simulink model "PVHome"  (R2022b)
settings: Solver=FixedStepDiscrete  StartTime=0.0  StopTime=2  FixedStep=5e-6  RelTol=1e-3
undefined symbols (not defined in the file): Ion, Lithium
libraries: spsSeriesRLCBranchLib x175, spsBreakerLib x103, spsPWMGeneratorDCDCLib x94, spsThyristorLib x78, slpidlib x72, spsIGBTDiodeLib x62, spsThreePhaseVIMeasurementLib x59, spsThreePhaseBreakerLib x45, spsVoltageMeasurementLib x45, spsDiodeLib x39, spsThreePhaseParallelRLCBranchLib x38, spsMosfetLib x32
(part 13 of 16)

== system PVHome/Subsystem6/Subsystem ==
  note: this must activate when no power is available in the pv or no sufficient power available in PV
  note: Buck conv
  note: REAL GRID
  note: House Load DC to AC conversion
  note: Buck conv
  note: Buck conv
  Add{1..4} (4 alike) : Sum  Inputs=+-
  Battery1 : spsBatteryLib/Battery  BatType=Lithium-Ion  ShowTempParam=off  ThermalPreset=no  ShowAgeParam=off  NomV=60  NomQ=50  SOC=50  Batt_Tr=1  PresetModel=off  MaxQ=50  MinV=45  FullV=69.8392  Dis_rate=21.7391  R=0.012  Normal_OP=45.2174  expZone="[64.8232      2.45652]"  current=[6.5 13 32.5]  Units=Time  Tci=20  NomT=20  T2=-30  MaxQ2=4.8  FullV2=7.1  Normal_OP2=5.655  expZone2="[6.58           1]"  Rca=0.6  ti=2000  Dp=0  Neq0=0  Tsim=1e6  Ta1=25  Qeol=5.4*0.9  Reol=0.013333*1.2  Char_age=[2.3478, 3]  Dis_age=[2.3478, 10]  N1=1500  N2=10500  N3=1000  N4=1400  Ta2=45  N5=950
  Breaker{11..13,17..18,20} (6 alike) : spsBreakerLib/Breaker  InitialState=0  SwitchingTimes="[1/60  5/60]"  External=on  BreakerResistance=0.01  SnubberResistance=1e6  SnubberCapacitance=inf  Measurements=None  MoreParameters=on  NoBreakLoop=off
  Bus Creator1 : BusCreator  Inputs=3
  Bus Selector2 : BusSelector  OutputSignals=SOC (%),Current (A),Voltage (V)
  CAPACITOR 15 : spsSeriesRLCBranchLib/Series RLC Branch  LConnTagsString=__new0  RConnTagsString=__new0  BranchType=RL  Resistance=1e-4  Inductance=1e-3  SetiL0=off  InitialCurrent=0  Capacitance=100e-6  Setx0=off  InitialVoltage=0  Measurements=None
  CAPACITOR 20 : spsSeriesRLCBranchLib/Series RLC Branch  LConnTagsString=__new0  RConnTagsString=__new0  BranchType=RC  Resistance=1e-4  Inductance=5e-3  SetiL0=off  InitialCurrent=0  Capacitance=100e-6  Setx0=off  InitialVoltage=0  Measurements=None
  CAPACITOR 21 : spsSeriesRLCBranchLib/Series RLC Branch  LConnTagsString=__new0  RConnTagsString=__new0  BranchType=RC  Resistance=1e-4  Inductance=5e-3  SetiL0=off  InitialCurrent=0  Capacitance=100e-6  Setx0=off  InitialVoltage=0  Measurements=None
  CAPACITOR 22 : spsSeriesRLCBranchLib/Series RLC Branch  LConnTagsString=__new0  RConnTagsString=__new0  BranchType=RL  Resistance=1e-4  Inductance=13e-3  SetiL0=off  InitialCurrent=0  Capacitance=100e-6  Setx0=off  InitialVoltage=0  Measurements=None
  CAPACITOR 27 : spsSeriesRLCBranchLib/Series RLC Branch  LConnTagsString=__new0  RConnTagsString=__new0  BranchType=RL  Resistance=1e-4  Inductance=1e-3  SetiL0=off  InitialCurrent=0  Capacitance=100e-6  Setx0=off  InitialVoltage=0  Measurements=None
  CAPACITOR 28 : spsSeriesRLCBranchLib/Series RLC Branch  LConnTagsString=__new0  RConnTagsString=__new0  BranchType=RC  Resistance=1e-4  Inductance=5e-3  SetiL0=off  InitialCurrent=0  Capacitance=2000e-3  Setx0=off  InitialVoltage=0  Measurements=None
  CAPACITOR 29 : spsSeriesRLCBranchLib/Series RLC Branch  LConnTagsString=__new0  RConnTagsString=__new0  BranchType=RC  Resistance=1e-4  Inductance=5e-3  SetiL0=off  InitialCurrent=0  Capacitance=2000e-3  Setx0=off  InitialVoltage=0  Measurements=None
  CAPACITOR 30 : spsSeriesRLCBranchLib/Series RLC Branch  LConnTagsString=__new0  RConnTagsString=__new0  BranchType=RL  Resistance=1e-4  Inductance=1e-3  SetiL0=off  InitialCurrent=0  Capacitance=100e-6  Setx0=off  InitialVoltage=0  Measurements=None
  CAPACITOR 31 : spsSeriesRLCBranchLib/Series RLC Branch  LConnTagsString=__new0  RConnTagsString=__new0  BranchType=RC  Resistance=1e-4  Inductance=5e-3  SetiL0=off  InitialCurrent=0  Capacitance=2000e-3  Setx0=off  InitialVoltage=0  Measurements=None
  Constant7 : Constant  Value=60
  Constant9 : Constant  Value=2300
  Current Measurement4 : spsCurrentMeasurementLib/Current Measurement  PhasorSimulation=off  OutputType=Complex  PSBequivalent=0
  Data Type Conversion3 : DataTypeConversion  OutDataTypeStr=boolean  SaturateOnIntegerOverflow=off  RndMeth=Floor
  Demux1 : Demux  Outputs=2
  Diode5 : spsDiodeLib/Diode  Ron=0.001  Lon=0  Vf=0.8  IC=0  UseSnubber=0  Rs=500  Cs=250e-9  Measurements=off
  Diode7 : spsDiodeLib/Diode  Ron=0.001  Lon=0  Vf=0.8  IC=0  UseSnubber=0  Rs=500  Cs=250e-9  Measurements=off
  Discrete PID Controller1 : slpidlib/PID Controller  Controller=PI  Form=Parallel  TimeDomain=Discrete-time  UseExternalTs=off  SampleTime=1e-5  IntegratorMethod=Forward Euler  FilterMethod=Forward Euler  ControllerParametersSource=internal  P=0  I=0.01  UseKiTs=off  D=0  N=100  UseFilter=on  TunerSelectOption=Transfer Function Based (PID Tuner App)  InitialConditionSource=internal  InitialConditionForIntegrator=0  InitialConditionForFilter=0  DifferentiatorICPrevScaledInput=0  ExternalReset=none  TrackingMode=off  Kt=1  LimitOutput=on  SatLimitsSource=internal  UpperSaturationLimit=1.1  LowerSaturationLimit=-1.1  LinearizeAsGain=off  AntiWindupMode=none  Kb=1  LimitIntegrator=off  UpperIntegratorSaturationLimit=inf  LowerIntegratorSaturationLimit=-inf  POutMin=[]  POutMax=[]  IOutMin=[]  IOutMax=[]  DOutMin=[]  DOutMax=[]  NOutMin=[]  NOutMax=[]  SumOutMin=[]  SumOutMax=[]  SaturationOutMin=[]  SaturationOutMax=[]  PParamMin=[]  PParamMax=[]  IParamMin=[]  IParamMax=[]  DParamMin=[]  DParamMax=[]  NParamMin=[]  NParamMax=[]  KbParamMin=[]  KbParamMax=[]  KtParamMin=[]  KtParamMax=[]  KbOutMin=[]  KbOutMax=[]  KtOutMin=[]  KtOutMax=[]  IntegratorOutMin=[]  IntegratorOutMax=[]  FilterOutMin=[]  FilterOutMax=[]  SumI1OutMin=[]  SumI1OutMax=[]  SumI2OutMin=[]  SumI2OutMax=[]  SumI3OutMin=[]  SumI3OutMax=[]  SumI4OutMin=[]  SumI4OutMax=[]  SumDOutMin=[]  SumDOutMax=[]  DifferentiatorOutMin=[]  DifferentiatorOutMax=[]  FilterDiffOutCoefMin=[]  FilterDiffOutCoefMax=[]  ReciprocalOutMin=[]  ReciprocalOutMax=[]  SumDenOutMin=[]  SumDenOutMax=[]  SumNumOutMin=[]  SumNumOutMax=[]  DivideOutMin=[]  DivideOutMax=[]  UdiffTsProdOutMin=[]  UdiffTsProdOutMax=[]  NTsProdOutMin=[]  NTsProdOutMax=[]  UintegralTsProdOutMin=[]  UintegralTsProdOutMax=[]  UngainTsProdOutMin=[]  UngainTsProdOutMax=[]  ClampingZeroOutDataTypeStr=Inherit: Inherit via back propagation  ClampingZeroOutMin=[]  ClampingZeroOutMax=[]  FilterDenConstantOutDataTypeStr=Inherit: Inherit via back propagation  FilterDenConstantOutMin=[]  FilterDenConstantOutMax=[]  PCopyOutDataTypeStr=Inherit: Inherit via back propagation  PCopyOutMin=[]  PCopyOutMax=[]  NCopyOutDataTypeStr=Inherit: Inherit via back propagation  NCopyOutMin=[]  NCopyOutMax=[]  IntegratorContinuousStateAttributes=''  IntegratorStateMustResolveToSignalObject=off  IntegratorRTWStateStorageClass=Auto  FilterContinuousStateAttributes=''  FilterStateMustResolveToSignalObject=off  FilterRTWStateStorageClass=Auto  ParallelPVariant=InternalParameters  IdealPVariant=Disabled  IVariant=InternalParameters  DVariant=Disabled  IntegratorVariant=Discrete  SatVariant=Enabled  AWVariant=Passthrough  PCopyVariant=Disabled  TRVariant=Disabled  FdbkBlocksVariant=Forward  IdealPFdbkVariant=Disabled  SatFdbkVariant=Disabled  DerivativeFilterVariant=Disabled  NVariant=Disabled  NCopyVariant=Disabled_SignalSpec  FilterICVariant=Disabled  IntegratorICVariant=InternalICs  ExternalResetVariant=Disabled  TRSumVariant=Passthrough  SumFdbkVariant=Disabled  SumVariant=Sum_PI  TsampFilterVariant=InternalTs  TsampNgainVariant=Passthrough  TsampIntegralVariant=Passthrough  ExternalSaturationOutDataTypeStr=Inherit: Same as second input
      settings: LibrarySourceBlock=simulink/Discrete/Discrete PID Controller
  Discrete PID Controller2 : slpidlib/PID Controller  Controller=PI  Form=Parallel  TimeDomain=Discrete-time  UseExternalTs=off  SampleTime=1e-5  IntegratorMethod=Forward Euler  FilterMethod=Forward Euler  ControllerParametersSource=internal  P=0.01  I=1  UseKiTs=off  D=0  N=100  UseFilter=on  TunerSelectOption=Transfer Function Based (PID Tuner App)  InitialConditionSource=internal  InitialConditionForIntegrator=0  InitialConditionForFilter=0  DifferentiatorICPrevScaledInput=0  ExternalReset=none  TrackingMode=off  Kt=1  LimitOutput=on  SatLimitsSource=internal  UpperSaturationLimit=1.1  LowerSaturationLimit=-1.1  LinearizeAsGain=off  AntiWindupMode=none  Kb=1  LimitIntegrator=off  UpperIntegratorSaturationLimit=inf  LowerIntegratorSaturationLimit=-inf  POutMin=[]  POutMax=[]  IOutMin=[]  IOutMax=[]  DOutMin=[]  DOutMax=[]  NOutMin=[]  NOutMax=[]  SumOutMin=[]  SumOutMax=[]  SaturationOutMin=[]  SaturationOutMax=[]  PParamMin=[]  PParamMax=[]  IParamMin=[]  IParamMax=[]  DParamMin=[]  DParamMax=[]  NParamMin=[]  NParamMax=[]  KbParamMin=[]  KbParamMax=[]  KtParamMin=[]  KtParamMax=[]  KbOutMin=[]  KbOutMax=[]  KtOutMin=[]  KtOutMax=[]  IntegratorOutMin=[]  IntegratorOutMax=[]  FilterOutMin=[]  FilterOutMax=[]  SumI1OutMin=[]  SumI1OutMax=[]  SumI2OutMin=[]  SumI2OutMax=[]  SumI3OutMin=[]  SumI3OutMax=[]  SumI4OutMin=[]  SumI4OutMax=[]  SumDOutMin=[]  SumDOutMax=[]  DifferentiatorOutMin=[]  DifferentiatorOutMax=[]  FilterDiffOutCoefMin=[]  FilterDiffOutCoefMax=[]  ReciprocalOutMin=[]  ReciprocalOutMax=[]  SumDenOutMin=[]  SumDenOutMax=[]  SumNumOutMin=[]  SumNumOutMax=[]  DivideOutMin=[]  DivideOutMax=[]  UdiffTsProdOutMin=[]  UdiffTsProdOutMax=[]  NTsProdOutMin=[]  NTsProdOutMax=[]  UintegralTsProdOutMin=[]  UintegralTsProdOutMax=[]  UngainTsProdOutMin=[]  UngainTsProdOutMax=[]  ClampingZeroOutDataTypeStr=Inherit: Inherit via back propagation  ClampingZeroOutMin=[]  ClampingZeroOutMax=[]  FilterDenConstantOutDataTypeStr=Inherit: Inherit via back propagation  FilterDenConstantOutMin=[]  FilterDenConstantOutMax=[]  PCopyOutDataTypeStr=Inherit: Inherit via back propagation  PCopyOutMin=[]  PCopyOutMax=[]  NCopyOutDataTypeStr=Inherit: Inherit via back propagation  NCopyOutMin=[]  NCopyOutMax=[]  IntegratorContinuousStateAttributes=''  IntegratorStateMustResolveToSignalObject=off  IntegratorRTWStateStorageClass=Auto  FilterContinuousStateAttributes=''  FilterStateMustResolveToSignalObject=off  FilterRTWStateStorageClass=Auto  ParallelPVariant=InternalParameters  IdealPVariant=Disabled  IVariant=InternalParameters  DVariant=Disabled  IntegratorVariant=Discrete  SatVariant=Enabled  AWVariant=Passthrough  PCopyVariant=Disabled  TRVariant=Disabled  FdbkBlocksVariant=Forward  IdealPFdbkVariant=Disabled  SatFdbkVariant=Disabled  DerivativeFilterVariant=Disabled  NVariant=Disabled  NCopyVariant=Disabled_SignalSpec  FilterICVariant=Disabled  IntegratorICVariant=InternalICs  ExternalResetVariant=Disabled  TRSumVariant=Passthrough  SumFdbkVariant=Disabled  SumVariant=Sum_PI  TsampFilterVariant=InternalTs  TsampNgainVariant=Passthrough  TsampIntegralVariant=Passthrough  ExternalSaturationOutDataTypeStr=Inherit: Same as second input
      settings: LibrarySourceBlock=simulink/Discrete/Discrete PID Controller
  Discrete PID Controller3 : slpidlib/PID Controller  Controller=PI  Form=Parallel  TimeDomain=Discrete-time  UseExternalTs=off  SampleTime=1e-5  IntegratorMethod=Forward Euler  FilterMethod=Forward Euler  ControllerParametersSource=internal  P=0  I=0.01  UseKiTs=off  D=0  N=100  UseFilter=on  TunerSelectOption=Transfer Function Based (PID Tuner App)  InitialConditionSource=internal  InitialConditionForIntegrator=0  InitialConditionForFilter=0  DifferentiatorICPrevScaledInput=0  ExternalReset=none  TrackingMode=off  Kt=1  LimitOutput=on  SatLimitsSource=internal  UpperSaturationLimit=1.1  LowerSaturationLimit=-1.1  LinearizeAsGain=off  AntiWindupMode=none  Kb=1  LimitIntegrator=off  UpperIntegratorSaturationLimit=inf  LowerIntegratorSaturationLimit=-inf  POutMin=[]  POutMax=[]  IOutMin=[]  IOutMax=[]  DOutMin=[]  DOutMax=[]  NOutMin=[]  NOutMax=[]  SumOutMin=[]  SumOutMax=[]  SaturationOutMin=[]  SaturationOutMax=[]  PParamMin=[]  PParamMax=[]  IParamMin=[]  IParamMax=[]  DParamMin=[]  DParamMax=[]  NParamMin=[]  NParamMax=[]  KbParamMin=[]  KbParamMax=[]  KtParamMin=[]  KtParamMax=[]  KbOutMin=[]  KbOutMax=[]  KtOutMin=[]  KtOutMax=[]  IntegratorOutMin=[]  IntegratorOutMax=[]  FilterOutMin=[]  FilterOutMax=[]  SumI1OutMin=[]  SumI1OutMax=[]  SumI2OutMin=[]  SumI2OutMax=[]  SumI3OutMin=[]  SumI3OutMax=[]  SumI4OutMin=[]  SumI4OutMax=[]  SumDOutMin=[]  SumDOutMax=[]  DifferentiatorOutMin=[]  DifferentiatorOutMax=[]  FilterDiffOutCoefMin=[]  FilterDiffOutCoefMax=[]  ReciprocalOutMin=[]  ReciprocalOutMax=[]  SumDenOutMin=[]  SumDenOutMax=[]  SumNumOutMin=[]  SumNumOutMax=[]  DivideOutMin=[]  DivideOutMax=[]  UdiffTsProdOutMin=[]  UdiffTsProdOutMax=[]  NTsProdOutMin=[]  NTsProdOutMax=[]  UintegralTsProdOutMin=[]  UintegralTsProdOutMax=[]  UngainTsProdOutMin=[]  UngainTsProdOutMax=[]  ClampingZeroOutDataTypeStr=Inherit: Inherit via back propagation  ClampingZeroOutMin=[]  ClampingZeroOutMax=[]  FilterDenConstantOutDataTypeStr=Inherit: Inherit via back propagation  FilterDenConstantOutMin=[]  FilterDenConstantOutMax=[]  PCopyOutDataTypeStr=Inherit: Inherit via back propagation  PCopyOutMin=[]  PCopyOutMax=[]  NCopyOutDataTypeStr=Inherit: Inherit via back propagation  NCopyOutMin=[]  NCopyOutMax=[]  IntegratorContinuousStateAttributes=''  IntegratorStateMustResolveToSignalObject=off  IntegratorRTWStateStorageClass=Auto  FilterContinuousStateAttributes=''  FilterStateMustResolveToSignalObject=off  FilterRTWStateStorageClass=Auto  ParallelPVariant=InternalParameters  IdealPVariant=Disabled  IVariant=InternalParameters  DVariant=Disabled  IntegratorVariant=Discrete  SatVariant=Enabled  AWVariant=Passthrough  PCopyVariant=Disabled  TRVariant=Disabled  FdbkBlocksVariant=Forward  IdealPFdbkVariant=Disabled  SatFdbkVariant=Disabled  DerivativeFilterVariant=Disabled  NVariant=Disabled  NCopyVariant=Disabled_SignalSpec  FilterICVariant=Disabled  IntegratorICVariant=InternalICs  ExternalResetVariant=Disabled  TRSumVariant=Passthrough  SumFdbkVariant=Disabled  SumVariant=Sum_PI  TsampFilterVariant=InternalTs  TsampNgainVariant=Passthrough  TsampIntegralVariant=Passthrough  ExternalSaturationOutDataTypeStr=Inherit: Same as second input
      settings: LibrarySourceBlock=simulink/Discrete/Discrete PID Controller
  Discrete PID Controller6 : slpidlib/PID Controller  Controller=PI  Form=Parallel  TimeDomain=Discrete-time  UseExternalTs=off  SampleTime=-1  IntegratorMethod=Forward Euler  FilterMethod=Forward Euler  ControllerParametersSource=internal  P=1  I=1  UseKiTs=off  D=0  N=100  UseFilter=on  TunerSelectOption=Transfer Function Based (PID Tuner App)  InitialConditionSource=internal  InitialConditionForIntegrator=0  InitialConditionForFilter=0  DifferentiatorICPrevScaledInput=0  ExternalReset=none  TrackingMode=off  Kt=1  LimitOutput=off  SatLimitsSource=internal  UpperSaturationLimit=inf  LowerSaturationLimit=-inf  LinearizeAsGain=off  AntiWindupMode=none  Kb=1  LimitIntegrator=off  UpperIntegratorSaturationLimit=inf  LowerIntegratorSaturationLimit=-inf  POutMin=[]  POutMax=[]  IOutMin=[]  IOutMax=[]  DOutMin=[]  DOutMax=[]  NOutMin=[]  NOutMax=[]  SumOutMin=[]  SumOutMax=[]  SaturationOutMin=[]  SaturationOutMax=[]  PParamMin=[]  PParamMax=[]  IParamMin=[]  IParamMax=[]  DParamMin=[]  DParamMax=[]  NParamMin=[]  NParamMax=[]  KbParamMin=[]  KbParamMax=[]  KtParamMin=[]  KtParamMax=[]  KbOutMin=[]  KbOutMax=[]  KtOutMin=[]  KtOutMax=[]  IntegratorOutMin=[]  IntegratorOutMax=[]  FilterOutMin=[]  FilterOutMax=[]  SumI1OutMin=[]  SumI1OutMax=[]  SumI2OutMin=[]  SumI2OutMax=[]  SumI3OutMin=[]  SumI3OutMax=[]  SumI4OutMin=[]  SumI4OutMax=[]  SumDOutMin=[]  SumDOutMax=[]  DifferentiatorOutMin=[]  DifferentiatorOutMax=[]  FilterDiffOutCoefMin=[]  FilterDiffOutCoefMax=[]  ReciprocalOutMin=[]  ReciprocalOutMax=[]  SumDenOutMin=[]  SumDenOutMax=[]  SumNumOutMin=[]  SumNumOutMax=[]  DivideOutMin=[]  DivideOutMax=[]  UdiffTsProdOutMin=[]  UdiffTsProdOutMax=[]  NTsProdOutMin=[]  NTsProdOutMax=[]  UintegralTsProdOutMin=[]  UintegralTsProdOutMax=[]  UngainTsProdOutMin=[]  UngainTsProdOutMax=[]  ClampingZeroOutDataTypeStr=Inherit: Inherit via back propagation  ClampingZeroOutMin=[]  ClampingZeroOutMax=[]  FilterDenConstantOutDataTypeStr=Inherit: Inherit via back propagation  FilterDenConstantOutMin=[]  FilterDenConstantOutMax=[]  PCopyOutDataTypeStr=Inherit: Inherit via back propagation  PCopyOutMin=[]  PCopyOutMax=[]  NCopyOutDataTypeStr=Inherit: Inherit via back propagation  NCopyOutMin=[]  NCopyOutMax=[]  IntegratorContinuousStateAttributes=''  IntegratorStateMustResolveToSignalObject=off  IntegratorRTWStateStorageClass=Auto  FilterContinuousStateAttributes=''  FilterStateMustResolveToSignalObject=off  FilterRTWStateStorageClass=Auto  ParallelPVariant=InternalParameters  IdealPVariant=Disabled  IVariant=InternalParameters  DVariant=Disabled  IntegratorVariant=Discrete  SatVariant=Disabled  AWVariant=Passthrough  PCopyVariant=Disabled  TRVariant=Disabled  FdbkBlocksVariant=Forward  IdealPFdbkVariant=Disabled  SatFdbkVariant=Disabled  DerivativeFilterVariant=Disabled  NVariant=Disabled  NCopyVariant=Disabled_SignalSpec  FilterICVariant=Disabled  IntegratorICVariant=InternalICs  ExternalResetVariant=Disabled  TRSumVariant=Passthrough  SumFdbkVariant=Disabled  SumVariant=Sum_PI  TsampFilterVariant=InternalTs  TsampNgainVariant=Passthrough  TsampIntegralVariant=Passthrough  ExternalSaturationOutDataTypeStr=Inherit: Same as second input
      settings: LibrarySourceBlock=simulink/Discrete/Discrete PID Controller
  Discrete PID Controller7 : slpidlib/PID Controller  Controller=PI  Form=Parallel  TimeDomain=Discrete-time  UseExternalTs=off  SampleTime=1e-5  IntegratorMethod=Forward Euler  FilterMethod=Forward Euler  ControllerParametersSource=internal  P=0  I=0.01  UseKiTs=off  D=0  N=100  UseFilter=on  TunerSelectOption=Transfer Function Based (PID Tuner App)  InitialConditionSource=internal  InitialConditionForIntegrator=0  InitialConditionForFilter=0  DifferentiatorICPrevScaledInput=0  ExternalReset=none  TrackingMode=off  Kt=1  LimitOutput=on  SatLimitsSource=internal  UpperSaturationLimit=1.1  LowerSaturationLimit=-1.1  LinearizeAsGain=off  AntiWindupMode=none  Kb=1  LimitIntegrator=off  UpperIntegratorSaturationLimit=inf  LowerIntegratorSaturationLimit=-inf  POutMin=[]  POutMax=[]  IOutMin=[]  IOutMax=[]  DOutMin=[]  DOutMax=[]  NOutMin=[]  NOutMax=[]  SumOutMin=[]  SumOutMax=[]  SaturationOutMin=[]  SaturationOutMax=[]  PParamMin=[]  PParamMax=[]  IParamMin=[]  IParamMax=[]  DParamMin=[]  DParamMax=[]  NParamMin=[]  NParamMax=[]  KbParamMin=[]  KbParamMax=[]  KtParamMin=[]  KtParamMax=[]  KbOutMin=[]  KbOutMax=[]  KtOutMin=[]  KtOutMax=[]  IntegratorOutMin=[]  IntegratorOutMax=[]  FilterOutMin=[]  FilterOutMax=[]  SumI1OutMin=[]  SumI1OutMax=[]  SumI2OutMin=[]  SumI2OutMax=[]  SumI3OutMin=[]  SumI3OutMax=[]  SumI4OutMin=[]  SumI4OutMax=[]  SumDOutMin=[]  SumDOutMax=[]  DifferentiatorOutMin=[]  DifferentiatorOutMax=[]  FilterDiffOutCoefMin=[]  FilterDiffOutCoefMax=[]  ReciprocalOutMin=[]  ReciprocalOutMax=[]  SumDenOutMin=[]  SumDenOutMax=[]  SumNumOutMin=[]  SumNumOutMax=[]  DivideOutMin=[]  DivideOutMax=[]  UdiffTsProdOutMin=[]  UdiffTsProdOutMax=[]  NTsProdOutMin=[]  NTsProdOutMax=[]  UintegralTsProdOutMin=[]  UintegralTsProdOutMax=[]  UngainTsProdOutMin=[]  UngainTsProdOutMax=[]  ClampingZeroOutDataTypeStr=Inherit: Inherit via back propagation  ClampingZeroOutMin=[]  ClampingZeroOutMax=[]  FilterDenConstantOutDataTypeStr=Inherit: Inherit via back propagation  FilterDenConstantOutMin=[]  FilterDenConstantOutMax=[]  PCopyOutDataTypeStr=Inherit: Inherit via back propagation  PCopyOutMin=[]  PCopyOutMax=[]  NCopyOutDataTypeStr=Inherit: Inherit via back propagation  NCopyOutMin=[]  NCopyOutMax=[]  IntegratorContinuousStateAttributes=''  IntegratorStateMustResolveToSignalObject=off  IntegratorRTWStateStorageClass=Auto  FilterContinuousStateAttributes=''  FilterStateMustResolveToSignalObject=off  FilterRTWStateStorageClass=Auto  ParallelPVariant=InternalParameters  IdealPVariant=Disabled  IVariant=InternalParameters  DVariant=Disabled  IntegratorVariant=Discrete  SatVariant=Enabled  AWVariant=Passthrough  PCopyVariant=Disabled  TRVariant=Disabled  FdbkBlocksVariant=Forward  IdealPFdbkVariant=Disabled  SatFdbkVariant=Disabled  DerivativeFilterVariant=Disabled  NVariant=Disabled  NCopyVariant=Disabled_SignalSpec  FilterICVariant=Disabled  IntegratorICVariant=InternalICs  ExternalResetVariant=Disabled  TRSumVariant=Passthrough  SumFdbkVariant=Disabled  SumVariant=Sum_PI  TsampFilterVariant=InternalTs  TsampNgainVariant=Passthrough  TsampIntegralVariant=Passthrough  ExternalSaturationOutDataTypeStr=Inherit: Same as second input
      settings: LibrarySourceBlock=simulink/Discrete/Discrete PID Controller
  Divide{2,9..11} (4 alike) : Product  Inputs=**
  Ground2 : spsGroundLib/Ground  LConnTagsString=a
  IGBT/Diode{6..8,12} (4 alike) : spsIGBTDiodeLib/IGBT//Diode  Ron=1e-3  Rs=1e5  Cs=inf  Measurements=off
  MATLAB Function1 : MATLAB Function  TreatAsAtomicUnit=on
  MATLAB Function10 : MATLAB Function  TreatAsAtomicUnit=on
  MATLAB Function11 : MATLAB Function  TreatAsAtomicUnit=on
  MATLAB Function12 : MATLAB Function  TreatAsAtomicUnit=on
  MATLAB Function2 : MATLAB Function  TreatAsAtomicUnit=on
  MATLAB Function4 : MATLAB Function  TreatAsAtomicUnit=on
  MATLAB Function5 : MATLAB Function  TreatAsAtomicUnit=on
  MATLAB Function9 : MATLAB Function  TreatAsAtomicUnit=on
  Mosfet3 : spsMosfetLib/Mosfet  Ron=0.1  Lon=0  Rd=0.01  Vfd=0  IC=0  Rs=1e5  Cs=inf  Measurements=off
  Mosfet5 : spsMosfetLib/Mosfet  Ron=0.1  Lon=0  Rd=0.01  Vfd=0  IC=0  Rs=1e5  Cs=inf  Measurements=off
  Mux2 : Mux  Inputs=2
  NOT1 : Logic  Operator=NOT  IconShape=distinctive  AllPortsSameDT=off  OutDataTypeStr=boolean
  PF1 : Constant  Value=0.99
  PLL (3ph)1 : spsPLL3phLib/PLL (3ph)  Fmin=60  Par_Init=[0, 50]  ParK=[180, 3200, 1]  TcD=1e-4  MaxRateChangeFreq=12  FilterCutOffFreq=25  Ts=1e-5  AGC=on
  PWM Generator (2-Level)1 : spsPWMGenerator2LevelLib/PWM Generator (2-Level)  ModulatorType=Three-phase bridge (6 pulses)  ModulatorMode=Unsynchronized  Fc=27*60  Pc=90  nF=27  MinMax="[ -1  1 ]"  SamplingTechnique=Natural  ModulatingSignals=off  m=0.8  Freq=60  Phase=0  Ts=1e-5  ShowCarrierOutport=off
  PWM Generator (DC-DC){1..3,7..10} (7 alike) : spsPWMGeneratorDCDCLib/PWM Generator (DC-DC)  Fsw=10000  Ts=5e-6
  "Power (3ph, Instantaneous)1" : spsPower3phInstantaneousLib/Power (3ph, Instantaneous)
  Pulse Generator10 : DiscretePulseGenerator  PulseType=Time based  Period=0.02  PulseWidth=10  PhaseDelay=0*0.02/360
  Pulse Generator11 : DiscretePulseGenerator  PulseType=Time based  Period=0.02  PulseWidth=10  PhaseDelay=(0+180)*0.02/360
  Pulse Generator6 : DiscretePulseGenerator  PulseType=Time based  Period=0.02  PulseWidth=10  PhaseDelay=(0+60)*0.02/360
  Pulse Generator7 : DiscretePulseGenerator  PulseType=Time based  Period=0.02  PulseWidth=10  PhaseDelay=(0+120)*0.02/360
  Pulse Generator8 : DiscretePulseGenerator  PulseType=Time based  Period=0.02  PulseWidth=10  PhaseDelay=(0+240)*0.02/360
  Pulse Generator9 : DiscretePulseGenerator  PulseType=Time based  Period=0.02  PulseWidth=10  PhaseDelay=(0+360)*0.02/360
  Subtract3 : Sum  Inputs=+-
  Subtract4 : Sum  Inputs=+-
  Supply{1..6} (6 alike) : Constant  Value=60
  Three phase Inductor removes ripples4 : spsThreePhaseParallelRLCBranchLib/Three-Phase Parallel RLC Branch  LConnTagsString=A|B|C  RConnTagsString=A|B|C  BranchType=RL  Resistance=0.01  Inductance=1e-6  Capacitance=1e-6  Measurements=None
  Three phase Inductor removes ripples5 : spsThreePhaseParallelRLCBranchLib/Three-Phase Parallel RLC Branch  LConnTagsString=A|B|C  RConnTagsString=A|B|C  BranchType=RC  Resistance=0.01  Inductance=1e-6  Capacitance=1e-6  Measurements=None
  Three-Phase Series RLC Load1 : spsThreePhaseSeriesRLCLoadLib/Three-Phase Series RLC Load  LConnTagsString=A|B|C  Configuration=Y (grounded)  NominalVoltage=400  Vabc=[1e3 1e3 1e3]  Vabcp=[1e3 1e3 1e3]  NominalFrequency=60  UnbalancedPower=off  ActivePower=2300  InductivePower=1.5  CapacitivePower=0  Pabc=[10e3 9e3 11e3]  QLabc=[100 90 110]  QCabc=[100 90 110]  Pabcp=[10e3 9e3 11e3]  QLabcp=[100 90 110]  QCabcp=[100 90 110]  Measurements=Branch voltages and currents  LoadType=constant Z
  Three-Phase V-I Measurement5 : spsThreePhaseVIMeasurementLib/Three-Phase V-I Measurement  VoltageMeasurement=phase-to-ground  SetLabelV=on  LabelV=V_First  Vpu=off  VpuLL=off  CurrentMeasurement=yes  SetLabelI=on  LabelI=I_First  Ipu=off  Pbase=100e6  Vbase=500e3  OutputType=Complex  PhasorSimulation=off  PSBequivalent=0
  Three-Phase V-I Measurement6 : spsThreePhaseVIMeasurementLib/Three-Phase V-I Measurement  VoltageMeasurement=phase-to-ground  SetLabelV=on  LabelV=V_Real_Grid  Vpu=off  VpuLL=off  CurrentMeasurement=yes  SetLabelI=on  LabelI=I_Real_Grid  Ipu=off  Pbase=100e6  Vbase=500e3  OutputType=Complex  PhasorSimulation=off  PSBequivalent=0
  Three-Phase V-I Measurement7 : spsThreePhaseVIMeasurementLib/Three-Phase V-I Measurement  VoltageMeasurement=phase-to-ground  SetLabelV=on  LabelV=V_Real_Grid_Grid_C1  Vpu=off  VpuLL=off  CurrentMeasurement=yes  SetLabelI=on  LabelI=I_Real_Grid_Grid_C1  Ipu=off  Pbase=100e6  Vbase=500e3  OutputType=Complex  PhasorSimulation=off  PSBequivalent=0
  Three-Phase Breaker4 : spsThreePhaseBreakerLib/Three-Phase Breaker  InitialState=open  SwitchA=on  SwitchB=on  SwitchC=on  SwitchTimes="[1/50  10]"  External=on  BreakerResistance=0.01  SnubberResistance=1e6  SnubberCapacitance=inf  Measurements=None
  Three-Phase Breaker6 : spsThreePhaseBreakerLib/Three-Phase Breaker  InitialState=open  SwitchA=on  SwitchB=on  SwitchC=on  SwitchTimes="[1/50  10]"  External=on  BreakerResistance=0.01  SnubberResistance=1e6  SnubberCapacitance=inf  Measurements=None
  Thyristor{6..11} (6 alike) : spsThyristorLib/Thyristor  Ron=0.001  Lon=0  Vf=0.8  IC=0  Rs=500  Cs=250e-9  Measurements=off
  Trigonometric Function3 : Trigonometry  Operator=acos
  Trigonometric Function4 : Trigonometry
  Trigonometric Function5 : Trigonometry  Operator=cos
  Universal Bridge1 : spsUniversalBridgeLib/Universal Bridge  Arms=3  SnubberResistance=1e5  SnubberCapacitance=inf  Device=Thyristors  Ron=1e-3  Lon=0  ForwardVoltages="[  0  0  ]"  ForwardVoltage=0  GTOparameters=[ 10e-6 , 20e-6 ]  IGBTparameters=[ 1e-6 , 2e-6 ]  Measurements=None  Measurements_2=None  converterType=Rectifier
  Voltage Measurement5 : spsVoltageMeasurementLib/Voltage Measurement  PhasorSimulation=off  OutputType=Complex  PSBequivalent=0
  Voltage Measurement6 : spsVoltageMeasurementLib/Voltage Measurement  PhasorSimulation=off  OutputType=Complex  PSBequivalent=0
  kVAR1 : Gain  Gain=1/1000
  kW1 : Gain  Gain=1/1000
  a : PMIOPort  Side=Left
  + : PMIOPort  Port=2  Side=Left
  A1 : PMIOPort  Port=3  Side=Left
  B1 : PMIOPort  Port=4  Side=Left
  C1 : PMIOPort  Port=5  Side=Left
  wires:
  [V_PV_1] -> Add4/2
  [Buck_Prosumer] -> Mosfet3/1
  Voltage Measurement6/1 -> [V_Coming_Voltage_To_Battery]
  PWM Generator (DC-DC)7/1 -> NOT1/1, [P_H1_B]
  Discrete PID Controller2/1 -> Demux1/1
  [PWM_H1] -> Universal Bridge1/1
  Divide11/1 -> [P_Real_Grid_C1]
  [ma] -> MATLAB Function10/2(ma)
  Subtract4/1 -> [Q_Error]
  Pulse Generator6/1 -> Thyristor7/1
  [V_Consumer_Battery_Buck] -> Mosfet5/1
  MATLAB Function10/1(a) -> Bus Creator1/1
  MATLAB Function11/1(y) -> PWM Generator (DC-DC)10/1
  [V_Consumer_Battery_Buck_Breaker_Grid] -> Breaker18/1
  [P1_C1_Excess_C1_Control] -> Breaker20/1
  [V_Coming_Voltage_To_Battery] -> MATLAB Function5/3(V_Coming_Voltage_To_Battery)
  Pulse Generator8/1 -> Thyristor10/1
  Pulse Generator7/1 -> Thyristor11/1
  [Q_ref] -> Subtract4/1
  Supply4/1 -> Add4/1
  Divide10/1 -> [P_ref]
  kVAR1/1 -> [Q]
  Constant7/1 -> Add1/1
  [I_First] -> "Power (3ph, Instantaneous)1"/2
  Discrete PID Controller7/1 -> MATLAB Function11/1(u)
  Add1/1 -> Discrete PID Controller6/1
  Trigonometric Function3/1 -> Trigonometric Function4/1, Trigonometric Function5/1
  [wt] -> MATLAB Function10/1(x)
  Discrete PID Controller6/1 -> PWM Generator (DC-DC)7/1
  [Q] -> Subtract4/2
  Divide9/1 -> Divide2/1, Divide10/2
  Battery1/1 -> Bus Selector2/1
  Add4/1 -> Discrete PID Controller7/1
  [Grid_Battery_Switch] -> ?
  [P_Error] -> Mux2/1
  Current Measurement4/1 -> [I_Consumer_Current]
  [H1_Grid_Breaker] -> Data Type Conversion3/1
  [V_First] -> Divide9/1
  Pulse Generator10/1 -> Thyristor6/1
  PLL (3ph)1/2 -> [wt]
  kW1/1 -> [P]
  MATLAB Function5/4(H1_Battery_Discharge) -> [H1_Battery_Discharge]
  Supply3/1 -> MATLAB Function12/2(Sixty)
  "Power (3ph, Instantaneous)1"/2 -> kVAR1/1
  [N_H1_B] -> IGBT/Diode8/1
  Demux1/1 -> [ma]
  [V_PV_1] -> MATLAB Function12/1(V_PV_1)
  Demux1/2 -> [shift]
  MATLAB Function5/3(Grid_Battery_Switch) -> [Grid_Battery_Switch]
  [I_First] -> Divide9/2
  PF1/1 -> Trigonometric Function3/1
  Bus Selector2/3 -> [VbH1]  "<Voltage (V)>"
  Pulse Generator9/1 -> Thyristor8/1
  [V_Consumer_Battery_Boost_Breaker_Grid] -> Breaker17/1
  Bus Selector2/2 -> [IbH1]  "<Current (A)>"
  Bus Creator1/1 -> PWM Generator (2-Level)1/1
  MATLAB Function10/3(c) -> Bus Creator1/3
  [V_Consumer_Battery_Boost] -> IGBT/Diode12/1
  Pulse Generator11/1 -> Thyristor9/1
  MATLAB Function12/1(Wind_Breaker_Boost_Signal_Out) -> PWM Generator (DC-DC)9/1
  Bus Selector2/1 -> [SOCbHC1]  "<SOC (%)>"
  Voltage Measurement5/1 -> [V_Consumer_Battery]
  PWM Generator (2-Level)1/1 -> [PWM_H1]
  Mux2/1 -> Discrete PID Controller2/1
  [V_First] -> PLL (3ph)1/1
  [shift] -> MATLAB Function10/3(shift_k)
  [P_Real_Grid_C1] -> MATLAB Function5/6(P_Real_Grid_C1)
  Constant9/1 -> MATLAB Function5/5(Load)
  [V_Real_Grid_Grid_C1] -> Divide11/1
  "Power (3ph, Instantaneous)1"/1 -> kW1/1
  PWM Generator (DC-DC)10/1 -> [battery_buck_pwm]
  [Boost_From_The_Excess_Prosumer_Breaker] -> Breaker11/1
  [V_Consumer_Battery] -> MATLAB Function5/7(V_Consumer_Battery)
  [P_ref] -> Subtract3/1
  [Q_Error] -> Mux2/2
  Data Type Conversion3/1 -> ?
  [V_First] -> "Power (3ph, Instantaneous)1"/1
  MATLAB Function10/2(b) -> Bus Creator1/2
  [P_H1_B] -> IGBT/Diode7/1
  MATLAB Function5/6(Boost_From_The_Excess_Prosumer_Breaker) -> [Boost_From_The_Excess_Prosumer_Breaker]
  Trigonometric Function5/1 -> Divide10/1
  Subtract3/1 -> [P_Error]
  MATLAB Function5/1(V_Consumer_Battery_Boost_Breaker_Grid) -> [V_Consumer_Battery_Boost_Breaker_Grid]
  NOT1/1 -> [N_H1_B]
  [H1_Battery_Discharge] -> Breaker12/1
  [I_Real_Grid_Grid_C1] -> Divide11/2
  [P] -> Subtract3/2
  Divide2/1 -> [Q_ref]
  Trigonometric Function4/1 -> Divide2/2
  PWM Generator (DC-DC)9/1 -> [battery_boost_pwm]
  [IbH1] -> Add1/2
  [Buck_From_The_Excess_Prosumer_Breaker] -> Breaker13/1
  [P1_C1] -> MATLAB Function5/4(P1_C1)
  [V_PV_1] -> MATLAB Function5/2(V_PV_1)
  [SOCbHC1] -> MATLAB Function5/1(SOCbHC1)
  MATLAB Function5/2(V_Consumer_Battery_Buck_Breaker_Grid) -> [V_Consumer_Battery_Buck_Breaker_Grid]
  MATLAB Function5/5(Buck_From_The_Excess_Prosumer_Breaker) -> [Buck_From_The_Excess_Prosumer_Breaker]
  MATLAB Function5/7(P1_C1_Excess_C1_Control) -> [P1_C1_Excess_C1_Control]
  [Boost_Prosumer] -> IGBT/Diode6/1
  MATLAB Function4/1(y) -> PWM Generator (DC-DC)8/1
  Discrete PID Controller3/1 -> MATLAB Function4/1(u)
  Supply5/1 -> Add2/2
  Supply1/1 -> MATLAB Function9/1(Sixty)
  PWM Generator (DC-DC)3/1 -> [V_Consumer_Battery_Boost_Breaker_Grid]
  MATLAB Function9/1(Wind_Breaker_Boost_Signal_Out) -> PWM Generator (DC-DC)3/1
  [V_Consumer_Battery] -> MATLAB Function9/2(V_Consumer_Batter)
  Add2/1 -> Discrete PID Controller3/1
  [V_Consumer_Battery] -> Add2/1
  PWM Generator (DC-DC)8/1 -> [V_Consumer_Battery_Buck_Breaker_Grid]
  MATLAB Function2/1(Wind_Breaker_Boost_Signal_Out) -> PWM Generator (DC-DC)1/1
  Discrete PID Controller1/1 -> MATLAB Function1/1(u)
  MATLAB Function1/1(y) -> PWM Generator (DC-DC)2/1
  Add3/1 -> Discrete PID Controller1/1
  PWM Generator (DC-DC)1/1 -> [Boost_Prosumer]
  PWM Generator (DC-DC)2/1 -> [Buck_Prosumer]
  [V_Consumer_Battery] -> Add3/1
  [V_Consumer_Battery] -> MATLAB Function2/2(V_Consumer_Batter)
  Supply6/1 -> Add3/2
  Supply2/1 -> MATLAB Function2/1(Sixty)
  connections:
  Three-Phase Breaker4/LConn3 -- Three-Phase V-I Measurement6/LConn3 -- Three-Phase Breaker6/LConn3 -- Three-Phase V-I Measurement7/RConn3
  Three-Phase Breaker4/LConn2 -- Three-Phase V-I Measurement6/LConn2 -- Three-Phase Breaker6/LConn2 -- Three-Phase V-I Measurement7/RConn2
  CAPACITOR 21/LConn1 -- CAPACITOR 22/RConn1 -- Battery1/LConn1 -- Breaker12/LConn1
  Thyristor10/LConn1 -- Thyristor7/RConn1 -- Three-Phase Breaker6/RConn3
  CAPACITOR 15/RConn1 -- Diode5/LConn1 -- IGBT/Diode6/LConn1
  Diode7/RConn1 -- CAPACITOR 28/LConn1 -- Mosfet5/RConn1 -- CAPACITOR 20/LConn1 -- Diode5/RConn1 -- Mosfet3/RConn1 -- IGBT/Diode7/LConn1
  Three-Phase V-I Measurement7/LConn3 -- C1/RConn1
  Three-Phase V-I Measurement5/RConn3 -- Universal Bridge1/LConn3
  Three-Phase Breaker4/RConn3 -- Three-Phase V-I Measurement5/LConn3
  Three-Phase Breaker6/RConn1 -- Thyristor6/LConn1 -- Thyristor9/RConn1
  Voltage Measurement6/LConn2 -- Universal Bridge1/RConn2 -- Thyristor8/LConn1 -- Thyristor9/LConn1 -- Thyristor7/LConn1 -- CAPACITOR 29/RConn1 -- Voltage Measurement5/LConn2 -- CAPACITOR 31/RConn1 -- IGBT/Diode12/RConn1 -- CAPACITOR 28/RConn1 -- Battery1/LConn2 -- CAPACITOR 21/RConn1 -- IGBT/Diode8/RConn1 -- CAPACITOR 20/RConn1 -- IGBT/Diode6/RConn1 -- a/RConn1
  Three-Phase V-I Measurement7/LConn2 -- B1/RConn1
  Three phase Inductor removes ripples5/LConn3 -- Three phase Inductor removes ripples4/RConn3 -- Three-Phase Series RLC Load1/LConn3
  Three-Phase V-I Measurement6/RConn2 -- Three phase Inductor removes ripples4/LConn2
  CAPACITOR 30/RConn1 -- Current Measurement4/LConn1 -- Voltage Measurement5/LConn1
  Mosfet5/LConn1 -- Breaker18/RConn1
  CAPACITOR 29/LConn1 -- Thyristor10/RConn1 -- Thyristor6/RConn1 -- Thyristor11/RConn1 -- CAPACITOR 30/LConn1
  Thyristor11/LConn1 -- Thyristor8/RConn1 -- Three-Phase Breaker6/RConn2
  Breaker13/LConn1 -- Breaker20/RConn1 -- Breaker11/LConn1
  Three-Phase V-I Measurement7/RConn1 -- Three-Phase Breaker6/LConn1 -- Three-Phase Breaker4/LConn1 -- Three-Phase V-I Measurement6/LConn1
  Three-Phase Breaker4/RConn2 -- Three-Phase V-I Measurement5/LConn2
  Diode7/LConn1 -- CAPACITOR 27/RConn1 -- IGBT/Diode12/LConn1
  Voltage Measurement6/LConn1 -- Breaker20/LConn1 -- +/RConn1
  Three-Phase V-I Measurement6/RConn1 -- Three phase Inductor removes ripples4/LConn1
  Mosfet3/LConn1 -- Breaker13/RConn1
  CAPACITOR 22/LConn1 -- IGBT/Diode8/LConn1 -- IGBT/Diode7/RConn1
  CAPACITOR 31/LConn1 -- Breaker17/RConn1 -- CAPACITOR 27/LConn1
  Three-Phase Breaker4/RConn1 -- Three-Phase V-I Measurement5/LConn1
  Three-Phase V-I Measurement5/RConn2 -- Universal Bridge1/LConn2
  Breaker12/RConn1 -- Universal Bridge1/RConn1
  Current Measurement4/RConn1 -- Breaker18/LConn1 -- Breaker17/LConn1
  Three phase Inductor removes ripples5/LConn2 -- Three phase Inductor removes ripples4/RConn2 -- Three-Phase Series RLC Load1/LConn2
  Three phase Inductor removes ripples5/RConn1 -- Three phase Inductor removes ripples5/RConn3 -- Three phase Inductor removes ripples5/RConn2 -- Ground2/LConn1
  Three phase Inductor removes ripples4/RConn1 -- Three phase Inductor removes ripples5/LConn1 -- Three-Phase Series RLC Load1/LConn1
  Three-Phase V-I Measurement6/RConn3 -- Three phase Inductor removes ripples4/LConn3
  CAPACITOR 15/LConn1 -- Breaker11/RConn1
  Three-Phase V-I Measurement7/LConn1 -- A1/RConn1
  Three-Phase V-I Measurement5/RConn1 -- Universal Bridge1/LConn1

== system PVHome/Subsystem7/Subsystem ==
  In1 : Inport
  In2 : Inport  Port=2
  In3 : Inport  Port=3
  GreaterThan : RelationalOperator  OutDataTypeStr=boolean  RndMeth=Simplest  InputSameDT=off
  GreaterThan1 : RelationalOperator  OutDataTypeStr=boolean  RndMeth=Simplest  InputSameDT=off
  GreaterThan2 : RelationalOperator  OutDataTypeStr=boolean  RndMeth=Simplest  InputSameDT=off
  NOT : Logic  Operator=NOT  IconShape=distinctive  AllPortsSameDT=off  OutDataTypeStr=boolean
  NOT1 : Logic  Operator=NOT  IconShape=distinctive  AllPortsSameDT=off  OutDataTypeStr=boolean
  NOT2 : Logic  Operator=NOT  IconShape=distinctive  AllPortsSameDT=off  OutDataTypeStr=boolean
  Repeating Sequence : simulink/Sources/Repeating Sequence  rep_seq_t=[0 0.0001]  rep_seq_y=[-1 1]
  Out1 : Outport
  Out2 : Outport  Port=2
  Out3 : Outport  Port=3
  Out4 : Outport  Port=4
  Out5 : Outport  Port=5
  Out6 : Outport  Port=6
  wires:
  In1/1 -> GreaterThan/1
  In3/1 -> GreaterThan2/1
  In2/1 -> GreaterThan1/1
  Repeating Sequence/1 -> GreaterThan2/2, GreaterThan1/2, GreaterThan/2
  GreaterThan2/1 -> Out5/1, NOT2/1
  GreaterThan1/1 -> NOT1/1, Out3/1
  GreaterThan/1 -> Out1/1, NOT/1
  NOT2/1 -> Out6/1
  NOT1/1 -> Out4/1
  NOT/1 -> Out2/1

== matlab function PVHome/Subsystem3/Subsystem/MATLAB Function2 ==
  data: Sixty input; V_Consumer_Batter input; Wind_Breaker_Boost_Signal_Out output
function Wind_Breaker_Boost_Signal_Out = fcn(Sixty, V_Consumer_Batter)
Sixty = abs(Sixty);
V_Consumer_Batter = abs(V_Consumer_Batter);

D=1-(Sixty/V_Consumer_Batter);
Wind_Breaker_Boost_Signal_Out = D; %Vout

== matlab function PVHome/Subsystem3/Subsystem/MATLAB Function4 ==
  data: u input; y output
function y = fcn(u)
% This will output 1 - u
y = 1 - u;

== matlab function PVHome/Subsystem3/Subsystem/MATLAB Function9 ==
  data: Sixty input; V_Consumer_Batter input; Wind_Breaker_Boost_Signal_Out output
function Wind_Breaker_Boost_Signal_Out = fcn(Sixty, V_Consumer_Batter)
Sixty = abs(Sixty);
V_Consumer_Batter = abs(V_Consumer_Batter);

D=1-(Sixty/V_Consumer_Batter);
Wind_Breaker_Boost_Signal_Out = D; %Vout

== matlab function PVHome/Subsystem1/Subsystem/MATLAB Function1 ==
  data: u input; y output
function y = fcn(u)
% This will output 1 - u
y = 1 - u;

== matlab function PVHome/Subsystem1/Subsystem/MATLAB Function2 ==
  data: Sixty input; V_Consumer_Batter input; Wind_Breaker_Boost_Signal_Out output
function Wind_Breaker_Boost_Signal_Out = fcn(Sixty, V_Consumer_Batter)
Sixty = abs(Sixty);
V_Consumer_Batter = abs(V_Consumer_Batter);

D=1-(Sixty/V_Consumer_Batter);
Wind_Breaker_Boost_Signal_Out = D; %Vout

== matlab function PVHome/Subsystem1/Subsystem/MATLAB Function4 ==
  data: u input; y output
function y = fcn(u)
% This will output 1 - u
y = 1 - u;

== matlab function PVHome/Subsystem1/MATLAB Function ==
  data: V_PV input; duty output; I_PV input; deltaD input
function duty = mppt_pno(V_PV, I_PV, deltaD)

persistent prevP prevDuty

if isempty(prevP)
    prevP = 0;
    prevDuty = 0.5;   % Start at 50%
end

% Current PV power
P = V_PV * I_PV;

% Basic P&O
if P > prevP
    prevDuty = prevDuty + deltaD;
else
    prevDuty = prevDuty - deltaD;
end

% Safe duty limits for boost converter
if prevDuty > 0.75
    prevDuty = 0.75;
elseif prevDuty < 0.10
    prevDuty = 0.10;
end

% Update previous power
prevP = P;

% Output duty
duty = prevDuty;

end

== matlab function PVHome/Subsystem1/Subsystem/MATLAB Function9 ==
  data: Sixty input; V_Consumer_Batter input; Wind_Breaker_Boost_Signal_Out output
function Wind_Breaker_Boost_Signal_Out = fcn(Sixty, V_Consumer_Batter)
Sixty = abs(Sixty);
V_Consumer_Batter = abs(V_Consumer_Batter);

D=1-(Sixty/V_Consumer_Batter);
Wind_Breaker_Boost_Signal_Out = D; %Vout

== matlab function PVHome/Subsystem1/MATLAB Function5 ==
  data: Fault_Signal output; I_Fault input
function Fault_Signal = fcn(I_Fault)

I_Fault = abs(I_Fault)

Fault_Signal=0; %closed

if I_Fault>30
    Fault_Signal=1;
elseif I_Fault<30
    Fault_Signal=0;
end

== matlab function PVHome/Subsystem7/MATLAB Function ==
  data: Error input; Buck_Pwm output; Vdc input
function Buck_Pwm = fcn(Error, Vdc)
Error = abs(Error);
Vdc = abs(Vdc);

D=Error/Vdc;
Buck_Pwm = 1-D; %Vout

== matlab function PVHome/Subsystem7/MATLAB Function2 ==
  data: x input; a output size=1; ma input size=1; shift_k input size=1; b output; c output
function [a, b, c] = ref_generation(x, ma, shift_k)
  % x: electrical angle (rad), scalar
  % ma: modulation index, scalar
  % shift_k: phase offset angle, scalar
  a = ma * sin(x + shift_k);
  b = ma * sin(x + shift_k - 2*pi/3);
  c = ma * sin(x + shift_k + 2*pi/3);
end

== matlab function PVHome/MATLAB Function5 ==
  data: Fault_Signal output; I_Fault input
function Fault_Signal = fcn(I_Fault)

I_Fault = abs(I_Fault)

Fault_Signal=0; %closed

if I_Fault>30
    Fault_Signal=1;
elseif I_Fault<30
    Fault_Signal=0;
end

== matlab function PVHome/Subsystem/MATLAB Function1 ==
  data: u input; y output
function y = fcn(u)
% This will output 1 - u
y = 1 - u;

== matlab function PVHome/Subsystem/MATLAB Function10 ==
  data: x input; a output; ma input; shift_k input; b output; c output
function [a,b,c]=ref_generation(x,ma,shift_k)
a=(ma*(sin((x)+shift_k)));
b=(ma*(sin((x)+shift_k-(2*pi/3))));
c=(ma*(sin((x)+shift_k+(2*pi/3))));

%ma is modulation index
%x is wt rad/s
%shift_k is phase angle

== matlab function PVHome/Subsystem/MATLAB Function11 ==
  data: u input; y output
function y = fcn(u)
% This will output 1 - u
y = 1 - u;

== matlab function PVHome/Subsystem/MATLAB Function12 ==
  data: V_PV_1 input; Wind_Breaker_Boost_Signal_Out output; Sixty input
function Wind_Breaker_Boost_Signal_Out = fcn(V_PV_1, Sixty)
V_PV_1 = abs(V_PV_1);
Sixty = abs(Sixty);

D=1-(V_PV_1/Sixty);
Wind_Breaker_Boost_Signal_Out = D; %Vout

== matlab function PVHome/Subsystem/MATLAB Function2 ==
  data: Sixty input; V_Consumer_Batter input; Wind_Breaker_Boost_Signal_Out output
function Wind_Breaker_Boost_Signal_Out = fcn(Sixty, V_Consumer_Batter)
Sixty = abs(Sixty);
V_Consumer_Batter = abs(V_Consumer_Batter);

D=1-(Sixty/V_Consumer_Batter);
Wind_Breaker_Boost_Signal_Out = D; %Vout

== matlab function PVHome/Subsystem/MATLAB Function4 ==
  data: u input; y output
function y = fcn(u)
% This will output 1 - u
y = 1 - u;

== matlab function PVHome/Subsystem1/MATLAB Function1 ==
  data: u input
function export_live_data(u)
% export_live_data  MATLAB Function block that writes 4 signals live into Excel
% Input: u (4-element vector)
% Exact workbook path used: 'V:\IEEE\LIVEdata.xlsx'
%
% Structure preserved: all COM/workspace actions run via evalin('base', ...)

    coder.extrinsic('evalin','assignin','actxserver','datetime','char','warning');

    persistent initialized
    if isempty(initialized)
        initialized = false;
    end

    % Convert inputs to doubles
    a = double(u(1)); b = double(u(2)); c = double(u(3)); d = double(u(4));

    % Use an .xlsx workbook for live UI updates
    excelPath = 'V:\IEEE\LIVEdata.csv';

    % Initialization block executed once (all logic runs inside evalin strings)
    if ~initialized
        % Ensure Excel COM server exists in base workspace and open/create workbook
        evalin('base', [ ...
            'if ~exist(''excelApp'',''var'') || isempty(excelApp), ' ...
                'excelApp = actxserver(''Excel.Application''); excelApp.Visible = true; ' ...
            'end; ' ...
            'if exist(''' excelPath ''',''file'')==2, ' ...
                'wb = excelApp.Workbooks.Open(''' excelPath '''); ws = wb.Worksheets.Item(1); ' ...
            'else, ' ...
                'wb = excelApp.Workbooks.Add; ws = wb.Worksheets.Item(1); ' ...
                'ws.Range(''A1'').Value = ''Timestamp''; ws.Range(''B1'').Value = ''Signal1''; ' ...
                'ws.Range(''C1'').Value = ''Signal2''; ws.Range(''D1'').Value = ''Signal3''; ' ...
                'ws.Range(''E1'').Value = ''Signal4''; wb.SaveAs(''' excelPath '''); ' ...
            'end; ' ...
            'if ~exist(''excelRow'',''var'') || isempty(excelRow), ur = ws.UsedRange; excelRow = double(ur.Rows.Count) + 1; end;']);

        initialized = true;
    end

    % Create timestamp string using datetime (host MATLAB)
    ts = char(datetime('now', 'Format', 'yyyy-MM-dd HH:mm:ss.SSS'));

    % Pass values into base workspace temporary variables (RHS only)
    assignin('base', 'tmp_ts', ts);
    assignin('base', 'tmp_a', a);
    assignin('base', 'tmp_b', b);
    assignin('base', 'tmp_c', c);
    assignin('base', 'tmp_d', d);

    % Perform the worksheet write and force Excel UI update (all inside evalin)
    % Note: r is the row written; we save, increment excelRow, then force repaint and scroll.
    evalin('base', [ ...
        'r = excelRow; ' ...
        'ws.Range([''A'' num2str(r)]).Value = tmp_ts; ' ...
        'ws.Range([''B'' num2str(r)]).Value = tmp_a; ' ...
        'ws.Range([''C'' num2str(r)]).Value = tmp_b; ' ...
        'ws.Range([''D'' num2str(r)]).Value = tmp_c; ' ...
        'ws.Range([''E'' num2str(r)]).Value = tmp_d; ' ...
        'wb.Save; ' ...
        'excelRow = r + 1; ' ...
        'try, excelApp.ScreenUpdating = true; excelApp.Calculate; ' ...
             'if ~isempty(excelApp.ActiveWindow), excelApp.ActiveWindow.ScrollRow = r; end; ' ...
             'pause(0.02); ' ...
        'end;']);

end

== matlab function PVHome/Subsystem/MATLAB Function5 ==
  data: SOCbHC1 input; V_Consumer_Battery_Boost_Breaker_Grid output; V_Consumer_Battery_Buck_Breaker_Grid output; Grid_Battery_Switch output; V_PV_1 input; V_Coming_Voltage_To_Battery input; P1_C1 input; Load input; P_Real_Grid_C1 input; H1_Battery_Discharge output; Buck_From_The_Excess_Prosumer_Breaker output; Boost_From_The_Excess_Prosumer_Breaker output; V_Consumer_Battery input; P1_C1_Excess_C1_Control output
function [V_Consumer_Battery_Boost_Breaker_Grid,V_Consumer_Battery_Buck_Breaker_Grid, Grid_Battery_Switch, H1_Battery_Discharge, Buck_From_The_Excess_Prosumer_Breaker, Boost_From_The_Excess_Prosumer_Breaker, P1_C1_Excess_C1_Control] = fcn(SOCbHC1, V_PV_1, V_Coming_Voltage_To_Battery, P1_C1,Load, P_Real_Grid_C1, V_Consumer_Battery)


SOCbHC1 = abs(SOCbHC1);
V_PV_1 = abs(V_PV_1);
V_Consumer_Battery = abs(V_Consumer_Battery);
V_Coming_Voltage_To_Battery = abs(V_Coming_Voltage_To_Battery);
%V_Coming_Voltage_To_Battery will be equal to V_PV_1
P_Real_Grid_C1 = abs(P_Real_Grid_C1);

%%Default States
V_Consumer_Battery_Boost_Breaker_Grid=0;
V_Consumer_Battery_Buck_Breaker_Grid=0;
Grid_Battery_Switch=0; % AC switch, always closed. 0 means closed in here.
H1_Battery_Discharge=0;
Buck_From_The_Excess_Prosumer_Breaker=0;
Boost_From_The_Excess_Prosumer_Breaker=0;
P1_C1_Excess_C1_Control=0;

%%Case 1: Charge

if (SOCbHC1)<=90
    Grid_Battery_Switch=0;
    if (V_Consumer_Battery)>60
        V_Consumer_Battery_Buck_Breaker_Grid=1;
        V_Consumer_Battery_Boost_Breaker_Grid=0;
    elseif (V_Consumer_Battery)<60
        V_Consumer_Battery_Buck_Breaker_Grid=0;
        V_Consumer_Battery_Boost_Breaker_Grid=1;
    end

    if (P1_C1)==1 && (V_Coming_Voltage_To_Battery)>5
        P1_C1_Excess_C1_Control=1;
        if (V_Coming_Voltage_To_Battery)>60
            Buck_From_The_Excess_Prosumer_Breaker=1;
            Boost_From_The_Excess_Prosumer_Breaker=0;
        elseif (V_Coming_Voltage_To_Battery)<60
            Buck_From_The_Excess_Prosumer_Breaker=0;
            Boost_From_The_Excess_Prosumer_Breaker=1;
        end
    elseif (P1_C1)==0 && (V_Coming_Voltage_To_Battery)<5
        Buck_From_The_Excess_Prosumer_Breaker=0;
        Boost_From_The_Excess_Prosumer_Breaker=0;
        P1_C1_Excess_C1_Control=0;
    end

elseif (SOCbHC1)==90
    V_Consumer_Battery_Boost_Breaker_Grid=0;
    V_Consumer_Battery_Buck_Breaker_Grid=0;
    Grid_Battery_Switch=1;
    H1_Battery_Discharge=0;
    Buck_From_The_Excess_Prosumer_Breaker=0;
    Boost_From_The_Excess_Prosumer_Breaker=0;
    P1_C1_Excess_C1_Control=0;
end

%%Case 2 Discharge

if (Load> P_Real_Grid_C1) || P_Real_Grid_C1<100
    V_Consumer_Battery_Boost_Breaker_Grid=0;
    V_Consumer_Battery_Buck_Breaker_Grid=0;
    Grid_Battery_Switch=1; 
    H1_Battery_Discharge=1;
    Buck_From_The_Excess_Prosumer_Breaker=0;
    Boost_From_The_Excess_Prosumer_Breaker=0;
    P1_C1_Excess_C1_Control=0;
end

== matlab function PVHome/Subsystem/MATLAB Function9 ==
  data: Sixty input; V_Consumer_Batter input; Wind_Breaker_Boost_Signal_Out output
function Wind_Breaker_Boost_Signal_Out = fcn(Sixty, V_Consumer_Batter)
Sixty = abs(Sixty);
V_Consumer_Batter = abs(V_Consumer_Batter);

D=1-(Sixty/V_Consumer_Batter);
Wind_Breaker_Boost_Signal_Out = D; %Vout
